simulink model "LQR_EKF"  (R2024b)
settings: Solver=VariableStepAuto  StartTime=0.0  StopTime=tf  MaxStep=0.001  RelTol=1e-3
values from neighbouring files (symbols this model uses):
  C = [1 0 0 0; 0 0 1 0]    [Main_LQR_EKF.m]
  IC = [0 0 0 20]'    [Main_LQR_EKF.m]
  IC_obs = [0.2+IC(1), IC(2), IC(3)+0.001, IC(4)]'    [Main_LQR_EKF.m]
  ncurr_amp = 1e-2    (= 0.01)    [Main_LQR_EKF.m]
  npos_amp = 5e-2    (= 0.05)    [Main_LQR_EKF.m]
  nx = min(size(x_opt))    [Main_LQR_EKF.m]
  Qk = [1 0 0 0; 0 1 0 0; 0 0 1 0; 0 0 0 1]    [Main_LQR_EKF.m]
  Rk = [1 0; 0 10]    [Main_LQR_EKF.m]
  w_amp = 0.4e-2    (= 0.004)    [Main_LQR_EKF.m]
settings Model: Creator=nicvi  LastModifiedBy=nicvi

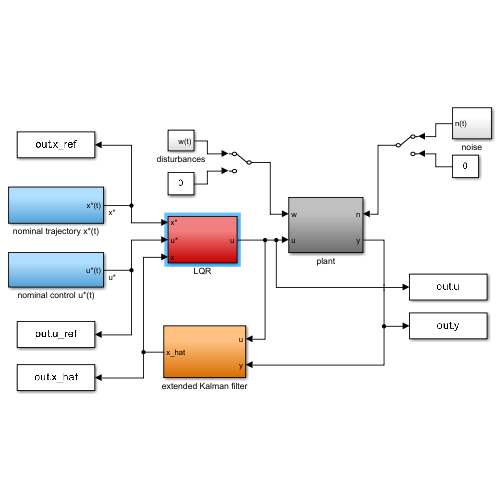
[thumbnail: Simulink's stored preview of the top-level diagram]
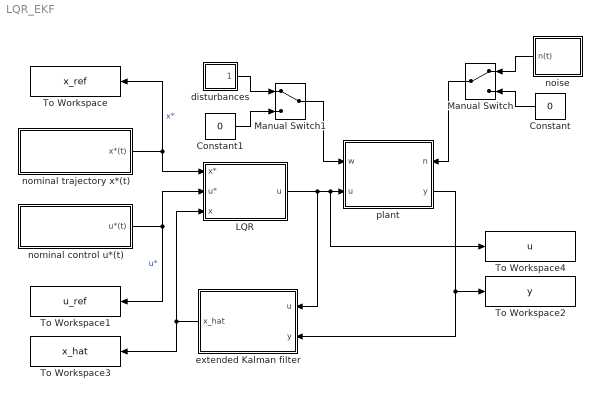
== system LQR_EKF ==
  Constant : Constant  Value=0
  Constant1 : Constant  Value=0
  LQR : Subsystem
  Manual Switch : ManualSwitch
  Manual Switch1 : ManualSwitch
  To Workspace : ToWorkspace  VariableName=x_ref  SampleTime=-1
      settings: Save2DSignal=2-D array (concatenate along first dimension)
  To Workspace1 : ToWorkspace  VariableName=u_ref  SampleTime=-1
      settings: Save2DSignal=2-D array (concatenate along first dimension)
  To Workspace2 : ToWorkspace  VariableName=y  SampleTime=-1
      settings: Save2DSignal=2-D array (concatenate along first dimension)
  To Workspace3 : ToWorkspace  VariableName=x_hat  SampleTime=-1
      settings: Save2DSignal=2-D array (concatenate along first dimension)
  To Workspace4 : ToWorkspace  VariableName=u  SampleTime=-1
      settings: Save2DSignal=2-D array (concatenate along first dimension)
  disturbances : Subsystem
  extended Kalman filter : Subsystem
  noise : Subsystem
      settings: PortSchema="{\"entries\":[{\"content\":{\"sides\":[{\"content\":{\"connectorIds\":[\"Out1\"]},\"type\":\"ConnectorPlacement.EquallySpacedRectSide\",\"uuid\":\"019152bc-1e26-4a91-b5d4-2b7e78122674\"},{\"content\":{\"side\":\"RIGHT\"},\"type\":\"ConnectorPlacement.EquallySpacedRectSide\",\"uuid\":\"b006df8a-a931-44a1-9c56-5e666493a0e5\"},{\"content\":{\"side\":\"TOP\"},\"type\":\"ConnectorPlacement.EquallySpacedRectSide\",\"uuid\":\"a8d284ac-8d56-4958-a6b1-f56e1b76591c\"}]},\"type\":\"ConnectorPlacement.EquallySpacedConnector\",\"uuid\":\"01c6f0d4-f763-43aa-add3-5ecb6e9648b4\"}],\"packageUris\":[\"http://schema.mathworks.com/mf0/Connector/R2020b\"],\"version\":\"1.0\"}"
  nominal control u*(t) : Subsystem
  nominal trajectory x*(t) : Subsystem
  plant : Subsystem
      settings: PortSchema="{\"entries\":[{\"content\":{\"sides\":[{\"content\":{\"connectorIds\":[\"In1\",\"In2\"]},\"type\":\"ConnectorPlacement.EquallySpacedRectSide\",\"uuid\":\"d558f5a9-0d92-4872-9cdb-75292574265c\"},{\"content\":{\"connectorIds\":[\"In3\",\"Out1\"],\"side\":\"RIGHT\"},\"type\":\"ConnectorPlacement.EquallySpacedRectSide\",\"uuid\":\"444b210a-d13a-4bc1-bb22-893f7af92ef0\"},{\"content\":{\"side\":\"TOP\"},\"type\":\"ConnectorPlacement.EquallySpacedRectSide\",\"uuid\":\"3e795392-0fce-42c0-8140-3cc224733c39\"}]},\"type\":\"ConnectorPlacement.EquallySpacedConnector\",\"uuid\":\"4c08022e-49cf-4277-8479-34c6b5d135b6\"}],\"packageUris\":[\"http://schema.mathworks.com/mf0/Connector/R2020b\"],\"version\":\"1.0\"}"
  wires:
  plant/1(y) -> To Workspace2/1, extended Kalman filter/2(y)
  Constant/1 -> Manual Switch/2
  nominal control u*(t)/1(u*(t)) -> To Workspace1/1, LQR/2(u*)  "u*"
  nominal trajectory x*(t)/1(x*(t)) -> To Workspace/1, LQR/1(x*)  "x*"
  noise/1(n(t)) -> Manual Switch/1
  Manual Switch/1 -> plant/3(n)
  extended Kalman filter/1(x_hat) -> To Workspace3/1, LQR/3(x)
  LQR/1(u) -> extended Kalman filter/1(u), To Workspace4/1, plant/2(u)
  Constant1/1 -> Manual Switch1/2
  disturbances/1(w(t)) -> Manual Switch1/1
  Manual Switch1/1 -> plant/1(w)

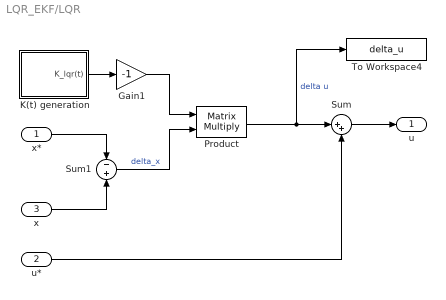
== system LQR_EKF/LQR ==
  x* : Inport
  u* : Inport  Port=2
  x : Inport  Port=3
  Gain1 : Gain  Gain=-1
  K(t) generation : Subsystem
  Product : Product  Multiplication=Matrix(*)
  Sum : Sum  Inputs=|++
  Sum1 : Sum  Inputs=-|+
  To Workspace4 : ToWorkspace  VariableName=delta_u  SampleTime=-1
      settings: Save2DSignal=2-D array (concatenate along first dimension)
  u : Outport
  wires:
  Product/1 -> To Workspace4/1, Sum/1  "delta u"
  u*/1 -> Sum/2
  Sum/1 -> u/1
  Sum1/1 -> Product/2  "delta_x"
  K(t) generation/1(K_lqr(t)) -> Gain1/1
  x*/1 -> Sum1/1
  x/1 -> Sum1/2
  Gain1/1 -> Product/1

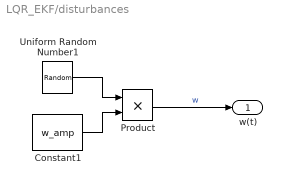
== system LQR_EKF/disturbances ==
  Constant1 : Constant  Value=w_amp  VectorParams1D=off
  Product : Product
  Uniform Random Number1 : UniformRandomNumber  Seed=143  SampleTime=tf/1000  VectorParams1D=off
  w(t) : Outport
  wires:
  Product/1 -> w(t)/1  "w"
  Constant1/1 -> Product/2
  Uniform Random Number1/1 -> Product/1

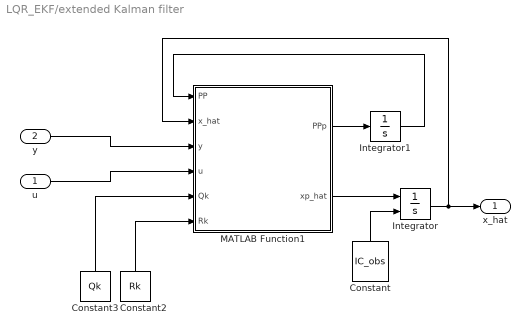
== system LQR_EKF/extended Kalman filter ==
  u : Inport
  y : Inport  Port=2
  Constant : Constant  Value=IC_obs
  Constant2 : Constant  Value=Rk
  Constant3 : Constant  Value=Qk
  Integrator : Integrator  InitialConditionSource=external
  Integrator1 : Integrator  InitialCondition=zeros(nx,nx)
  MATLAB Function1 : MATLAB Function  TreatAsAtomicUnit=on
  x_hat : Outport
  wires:
  MATLAB Function1/2(xp_hat) -> Integrator/1
  Constant/1 -> Integrator/2
  Integrator/1 -> MATLAB Function1/2(x_hat), x_hat/1
  MATLAB Function1/1(PPp) -> Integrator1/1
  Integrator1/1 -> MATLAB Function1/1(PP)
  u/1 -> MATLAB Function1/4(u)
  Constant3/1 -> MATLAB Function1/5(Qk)
  Constant2/1 -> MATLAB Function1/6(Rk)
  y/1 -> MATLAB Function1/3(y)

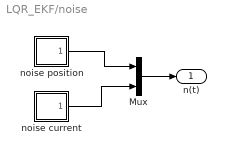
== system LQR_EKF/noise ==
  Mux : Mux  Inputs=2
  noise current : Subsystem
  noise position : Subsystem
  n(t) : Outport
  wires:
  noise position/1(n(t)) -> Mux/1
  Mux/1 -> n(t)/1
  noise current/1(n(t)) -> Mux/2

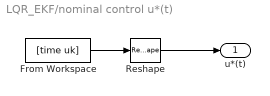
== system LQR_EKF/nominal control u*(t) ==
  From Workspace : FromWorkspace  VariableName=[time uk]
  Reshape : Reshape  OutputDimensionality=Column vector (2-D)
  u*(t) : Outport
  wires:
  Reshape/1 -> u*(t)/1
  From Workspace/1 -> Reshape/1

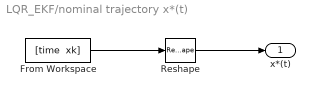
== system LQR_EKF/nominal trajectory x*(t) ==
  From Workspace : FromWorkspace  VariableName="[time  xk]"
  Reshape : Reshape  OutputDimensionality=Column vector (2-D)
  x*(t) : Outport
  wires:
  From Workspace/1 -> Reshape/1
  Reshape/1 -> x*(t)/1

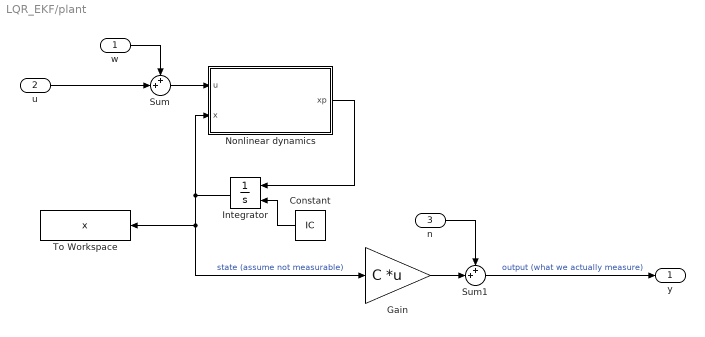
== system LQR_EKF/plant ==
  w : Inport
  u : Inport  Port=2
  n : Inport  Port=3
  Constant : Constant  Value=IC
  Gain : Gain  Gain=C  Multiplication=Matrix(K*u) (u vector)
  Integrator : Integrator  InitialConditionSource=external  InitialCondition=IC
  Nonlinear dynamics : MATLAB Function  TreatAsAtomicUnit=on
  Sum : Sum  Inputs=++|
  Sum1 : Sum  Inputs=++|
  To Workspace : ToWorkspace  VariableName=x  SampleTime=-1
      settings: Save2DSignal=2-D array (concatenate along first dimension)
  y : Outport
  wires:
  Nonlinear dynamics/1(xp) -> Integrator/1
  Constant/1 -> Integrator/2
  Gain/1 -> Sum1/2
  n/1 -> Sum1/1
  Sum1/1 -> y/1  "output (what we actually measure)"
  Integrator/1 -> Gain/1, To Workspace/1, Nonlinear dynamics/2(x)  "state (assume not measurable)"
  w/1 -> Sum/1
  Sum/1 -> Nonlinear dynamics/1(u)
  u/1 -> Sum/2

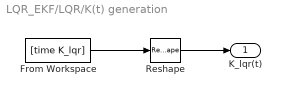
== system LQR_EKF/LQR/K(t) generation ==
  From Workspace : FromWorkspace  VariableName=[time K_lqr]
  Reshape : Reshape  OutputDimensionality=Row vector (2-D)
  K_lqr(t) : Outport
  wires:
  From Workspace/1 -> Reshape/1
  Reshape/1 -> K_lqr(t)/1

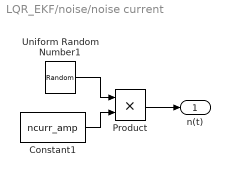
== system LQR_EKF/noise/noise current ==
  Constant1 : Constant  Value=ncurr_amp  VectorParams1D=off
  Product : Product
  Uniform Random Number1 : UniformRandomNumber  Seed=19  SampleTime=tf/500  VectorParams1D=off
  n(t) : Outport
  wires:
  Product/1 -> n(t)/1
  Uniform Random Number1/1 -> Product/1
  Constant1/1 -> Product/2

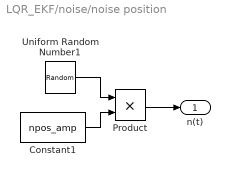
== system LQR_EKF/noise/noise position ==
  Constant1 : Constant  Value=npos_amp  VectorParams1D=off
  Product : Product
  Uniform Random Number1 : UniformRandomNumber  Seed=19  SampleTime=tf/500  VectorParams1D=off
  n(t) : Outport
  wires:
  Product/1 -> n(t)/1
  Uniform Random Number1/1 -> Product/1
  Constant1/1 -> Product/2

== matlab function LQR_EKF/plant/Nonlinear dynamics ==
  data: u input; x input; xp output
function xp=EquationOfMotion(u,x)

% parameters

m=0.5;          % mass of the piston [kg]
c=1;         % damping [N s/m]
k1=1;           % stiffness coefficient [N/m]
k3=0.1;         % stiffness coefficient [N/m^3]
alpha=50;       % force constant [N/A]
L0=0.1;         % inductance at reference temperature [H]
beta1=-7e-5;    % inductance coefficient [H/°C]
beta2=2e-7;     % inductance coefficient [H/°C^2]
RES=10;         % resistance [Ohm]
Ct=500;         % thermal capacity [J/°C]
h=10;           % thermal dissipation coefficient [W/°C]
Ta=20;          % ambient temperature [°C]

% differential equation of motion

xp=zeros(4,1);

xp(1)=x(2);
xp(2)=-k1/m*x(1)-k3/m*x(1)^3-c/m*x(2)+alpha/m*x(3);
xp(3)=-RES/(L0+beta1*x(4)+beta2*x(4)^2)*x(3)+u/(L0+beta1*x(4)+beta2*x(4)^2);
xp(4)=1/Ct*(RES*x(3)^2-h*(x(4)-Ta));

end

== matlab function LQR_EKF/extended Kalman filter/MATLAB Function1 ==
  data: PP input; PPp output; x_hat input; y input; xp_hat output; u input; Qk input; Rk input
function [PPp,xp_hat]=EKF(PP,x_hat,y,u,Qk,Rk)

% parameters and data

m=0.5;          % mass of the piston [kg]
c=1;         % damping [N s/m]
k1=1;           % stiffness coefficient [N/m]
k3=0.1;         % stiffness coefficient [N/m^3]
alpha=50;       % force constant [N/A]
L0=0.1;         % inductance at reference temperature [H]
beta1=-7e-5;    % inductance coefficient [H/°C]
beta2=2e-7;     % inductance coefficient [H/°C^2]
RES=10;         % resistance [Ohm]
Ct=500;         % thermal capacity [J/°C]
h_diss=10;      % thermal dissipation coefficient [W/°C]
Ta=20;          % ambient temperature [°C]

C=[1 0 0 0; 0 0 1 0];                                                              % output matrix (defines what are the outputs we are measuring)

f=@(x,u) [x(2);                                                                    % nonlinear model of the system - dynamics
          -k1/m*x(1)-k3/m*x(1)^3-c/m*x(2)+alpha/m*x(3);
          -RES/(L0+beta1*x(4)+beta2*x(4)^2)*x(3)+u/(L0+beta1*x(4)+beta2*x(4)^2);
          1/Ct*(RES*x(3)^2-h_diss*(x(4)-Ta))];  

h=@(x) C*x;                                                                        % nonlinear model of the system - output equation

% linearisation around the extimated state

A_xhat=[          0,               1,                  0,                                                  0;                                    % A_xhat = dfdx|x_hat,u
        -(k1+3*k3*x_hat(1)^2)/m, -c/m,              alpha/m,                                               0;
                  0,               0,   -RES/(L0+beta1*x_hat(4)+beta2*x_hat(4)^2), ((RES*x_hat(3)-u)*(beta1+2*beta2*x_hat(4)))/(L0+beta1*x_hat(4)+beta2*x_hat(4)^2)^2;
                  0,               0,             2*RES*x_hat(3)/Ct,                                    -h_diss/Ct                                                    ];

C_xhat=C;                                           % C_xhat = dhdx|x_hat,u

L_xhat=zeros(4);                                    % L_xhat = dfdw|x_hat,u (! say uncertainities enter with u in f3)
L_xhat(3,3)=1/(L0+beta1*x_hat(4)+beta2*x_hat(4)^2);    

M_xhat=[1 1];                                       % M_xhat = dhdv|x_hat,u

% differential Riccati equation (PP is the (nx,nx) Riccati matrix)

PPp=A_xhat*PP+PP*A_xhat'+L_xhat*Qk*L_xhat'-PP*C_xhat'*inv(M_xhat*Rk*M_xhat')*C_xhat*PP;

% Kalman gain equation

K_obs=PP*C_xhat'*inv(M_xhat*Rk*M_xhat');

% filter equation

xp_hat=f(x_hat,u)+K_obs*(y-h(x_hat));

end
